simulink model "flightControlSystem"  (R2022b)
settings: Solver=ode3  StartTime=0  StopTime=TFinal  FixedStep=Ts  RelTol=1e-3  EnableMultiTasking=on
model workspace (MAT data in the model file):
  D_gain = 0.03
  I_gain = 1.9
  PD_gain = 4e-05
  P_gain = 6
  case0_gain = 0.999
  en = 0.4
  kado_delay = 20
  last_gain = 0.0008
  ririku = 400
  start = 1400
undefined symbols (not defined in the file): codertarget, Controller, DiscIntNeverNeededParam, Discrete, Estimator, g, gray, init, Sensors, Time, Ts, var_acc_angle_N, var_bias_gyr_N, var_gyro_p_N, Vehicle
libraries: simulink x80, visionstatistics x8, sldvlib x7, slpidlib x4, ctrlSharedLib x4, sharedtransform x3, dspstat3 x2, parrotlib x1
(part 1 of 3)
settings Model: ExtModeTrigDuration=80  Creator=The MathWorks, Inc.  LastModifiedBy=yasuh
settings SolverCC: ZeroCrossControl=DisableAll  AlgebraicLoopSolver=TrustRegion
settings DataIOCC: LimitDataPoints=on  SaveFormat=StructureWithTime  SaveOutput=off  DSMLogging=off  SaveTime=off  ReturnWorkspaceOutputs=off
settings OptimizationCC: BlockReduction=off  EnhancedBackFolding=on  PassReuseOutputArgsThreshold=0  MaxStackSize=64  OptimizeBlockOrder=speed  DifferentSizesBufferReuse=on  OptimizationCustomize=off
settings DebuggingCC: AlgebraicLoopMsg=none  ParameterPrecisionLossMsg=none  ParameterTunabilityLossMsg=error  BusObjectLabelMismatch=error  PregeneratedLibrarySubsystemCodeDiagnostic=none  SFUnexpectedBacktrackingDiag=warning  SFNoUnconditionalDefaultTransitionDiag=warning  SFExecutionAtInitializationDiag=none  SFMachineParentedDataDiag=warning  ArithmeticOperatorsInVariantConditions=warning
settings HardwareCC: ProdBitPerPointer=32  ProdBitPerSizeT=32  ProdBitPerPtrDiffT=32  ProdLargestAtomicInteger=Long  ProdWordSize=32  ProdHWDeviceType=ARM Compatible->ARM 9  UseEmbeddedCoderFeatures=off  UseSimulinkCoderFeatures=off
settings ModelReferenceCC: EnableRefExpFcnMdlSchedulingChecks=on  ModelReferenceNumInstancesAllowed=Single  PropagateSignalLabelsOutOfModel=off
settings SFSimCC: SimUseLocalCustomCode=off  MATLABDynamicMemAlloc=off  CustomCodeUndefinedFunction=UseInterfaceOnly
settings RTWCC: Description=Embedded Coder  SystemTargetFile=ert.tlc  HardwareBoard=PARROT Mambo  TLCOptions=-aInlineSetEventsForThisBaseRateFcn=TLC_FALSE -aSuppressMultiTaskScheduler=TLC_FALSE -aRateBasedStepFcn=1  TemplateMakefile=ert_default_tmf  RTWUseLocalCustomCode=off  Toolchain=Sourcery G++ Lite GNU Toolchain for Drones  DLArmComputeVersion=19.05
settings CodeAppCC: ForceParamTrailComments=on  MaxIdLength=63  OperatorAnnotations=on
settings ERTTargetCC: CombineOutputUpdateFcns=off  ERTCustomFileBanners=off  SupportContinuousTime=on  SupportNonInlinedSFcns=on  RemoveResetFunc=off  ModelStepFunctionPrototypeControlCompliant=off
settings ConfigComp: CovMetricSettings=dw  CovSaveCumulativeToWorkspaceVar=on  CovSaveSingleToWorkspaceVar=on  CovExternalEMLEnable=off  CovSFcnEnable=off

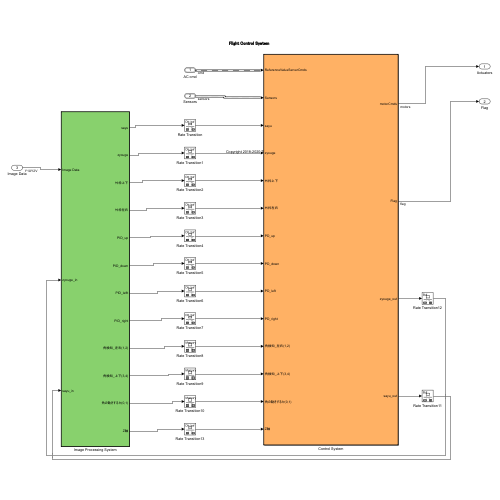
[thumbnail: Simulink's stored preview of the top-level diagram]
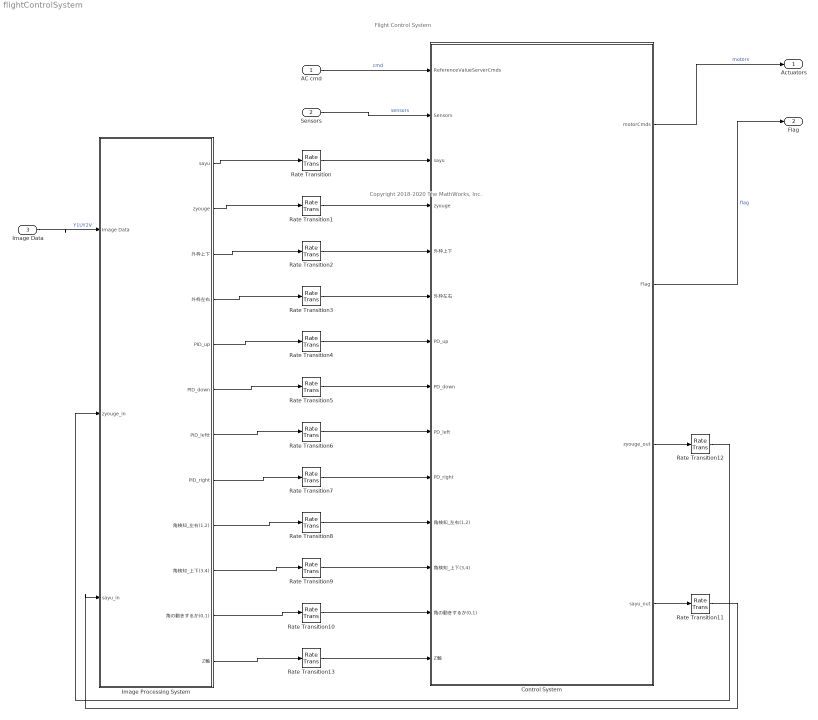
== system flightControlSystem ==
  note: Copyright 2018-2020 The MathWorks, Inc.
  note: Flight Control System
  AC cmd : Inport  OutDataTypeStr=Bus: CommandBus  BusOutputAsStruct=on
  Sensors : Inport  Port=2  OutDataTypeStr=Bus: SensorsBus  BusOutputAsStruct=on
  Image Data : Inport  Tag=IP_IN  InitFcn=codertarget.parrot.internal.inportCallback(gcb);  Port=3  OutDataTypeStr=uint8  PortDimensions=[4 9600]  BusOutputAsStruct=on
  Control System : Subsystem  InitFcn=codertarget.parrot.internal.fcsSubsystemCallback(gcb);  TreatAsAtomicUnit=on  SystemSampleTime=Ts
  Image Processing System : Subsystem  Tag=IP_SUB  InitFcn=codertarget.parrot.internal.ipSubsystemCallback(gcb);  TreatAsAtomicUnit=on  SystemSampleTime=40*Ts  RTWFcnName=ImageFunction
      settings: RTWSystemCode=Inline  RTWFcnNameOpts=User specified
  Rate Transition{,1..13} (14 alike) : RateTransition  Deterministic=off
  Actuators : Outport  OutDataTypeStr=single  PortDimensions=4  VectorParamsAs1DForOutWhenUnconnected=off
  Flag : Outport  Port=2  OutDataTypeStr=uint8  PortDimensions=1  VectorParamsAs1DForOutWhenUnconnected=off
  wires:
  AC cmd/1 -> Control System/1(ReferenceValueServerCmds)  "cmd"
  Control System/1(motorCmds) -> Actuators/1  "motors"
  Sensors/1 -> Control System/2(Sensors)  "sensors"
  Control System/2(Flag) -> Flag/1  "flag"
  Image Data/1 -> Image Processing System/1(Image Data)  "Y1UY2V"
  Image Processing System/1(sayu) -> Rate Transition/1
  Rate Transition/1 -> Control System/3(sayu)
  Image Processing System/2(zyouge) -> Rate Transition1/1
  Rate Transition1/1 -> Control System/4(zyouge)
  Image Processing System/3(外枠上下) -> Rate Transition2/1
  Image Processing System/4(外枠左右) -> Rate Transition3/1
  Rate Transition2/1 -> Control System/5(外枠上下)
  Rate Transition3/1 -> Control System/6(外枠左右)
  Image Processing System/5(PID_up) -> Rate Transition4/1
  Image Processing System/6(PID_down) -> Rate Transition5/1
  Rate Transition4/1 -> Control System/7(PD_up)
  Rate Transition5/1 -> Control System/8(PD_down)
  Image Processing System/7(PID_leftt) -> Rate Transition6/1
  Image Processing System/8(PID_right) -> Rate Transition7/1
  Rate Transition6/1 -> Control System/9(PD_left)
  Rate Transition7/1 -> Control System/10(PD_right)
  Image Processing System/11(角の動きするか(0,1)) -> Rate Transition10/1
  Rate Transition10/1 -> Control System/13(角の動きするか(0,1))
  Image Processing System/10(角検知_上下(3,4)) -> Rate Transition9/1
  Image Processing System/9(角検知_左右(1,2)) -> Rate Transition8/1
  Rate Transition9/1 -> Control System/12(角検知_上下(3,4))
  Rate Transition8/1 -> Control System/11(角検知_左右(1,2))
  Control System/3(zyouge_out) -> Rate Transition12/1
  Control System/4(sayu_out) -> Rate Transition11/1
  Rate Transition12/1 -> Image Processing System/2(zyouge_in)
  Rate Transition11/1 -> Image Processing System/3(sayu_in)
  Rate Transition13/1 -> Control System/14(Z軸)
  Image Processing System/12(Z軸) -> Rate Transition13/1

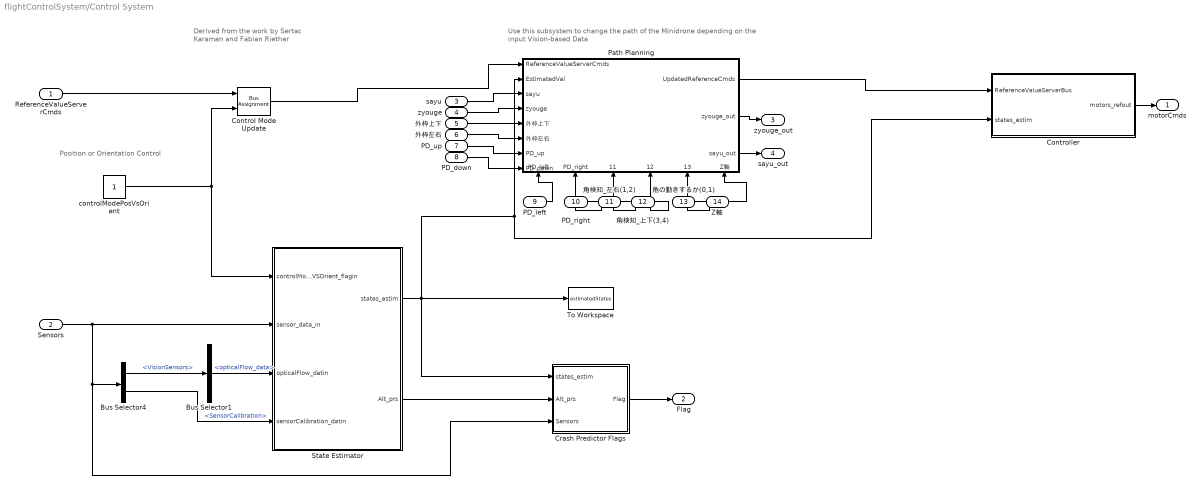
== system flightControlSystem/Control System ==
  note: Position or Orientation Control
  note: Use this subsystem to change the path of the
      | Minidrone depending on the input Vision-based
      | Data
  note: Derived from the work by Sertac
      | Karaman and Fabian Riether
  ReferenceValueServerCmds : Inport  OutDataTypeStr=Bus: CommandBus
  Sensors : Inport  Port=2  OutDataTypeStr=Bus: SensorsBus  BusOutputAsStruct=on
  sayu : Inport  Port=3
  zyouge : Inport  Port=4
  外枠上下 : Inport  Port=5
  外枠左右 : Inport  Port=6
  PD_up : Inport  Port=7
  PD_down : Inport  Port=8
  PD_left : Inport  Port=9
  PD_right : Inport  Port=10
  角検知_左右(1,2) : Inport  Port=11
  角検知_上下(3,4) : Inport  Port=12
  角の動きするか(0,1) : Inport  Port=13
  Z軸 : Inport  Port=14
  Bus Selector1 : BusSelector  OutputSignals=opticalFlow_data
  Bus Selector4 : BusSelector  OutputSignals=VisionSensors,SensorCalibration
  Control Mode Update : BusAssignment  AssignedSignals=controlModePosVSOrient
  Controller : Subsystem
  Crash Predictor Flags : Subsystem
  Path Planning : Subsystem
      settings: PortSchema="{\"entries\":[{\"content\":{\"sides\":[{\"content\":{\"connectorIds\":[\"In1\",\"In2\",\"In3\",\"In4\",\"In5\",\"In6\",\"In7\",\"In8\"]},\"type\":\"ConnectorPlacement.EquallySpacedRectSide\",\"uuid\":\"efe67c61-e99a-4cd7-b5d7-47091d682307\"},{\"content\":{\"connectorIds\":[\"Out1\",\"Out2\",\"Out3\"],\"side\":\"RIGHT\"},\"type\":\"ConnectorPlacement.EquallySpacedRectSide\",\"uuid\":\"b5496404-cc03-4446-9fbd-bd02e24f55c4\"},{\"content\":{\"connectorIds\":[],\"side\":\"TOP\"},\"type\":\"ConnectorPlacement.EquallySpacedRectSide\",\"uuid\":\"cc2bfd9b-f440-461f-8dfc-c1236b38a8d6\"},{\"content\":{\"connectorIds\":[\"In9\",\"In10\",\"In11\",\"In12\",\"In13\",\"In14\"],\"side\":\"BOTTOM\"},\"type\":\"ConnectorPlacement.EquallySpacedRectSide\",\"uuid\":\"b1dd3da0-6104-42b8-85e5-4e9639fd54d3\"}]},\"type\":\"ConnectorPlacement.EquallySpacedConnector\",\"uuid\":\"29da74a2-0098-4abc-a5c4-0db84ec285cd\"}],\"packageUris\":[\"http://schema.mathworks.com/mf0/Connector/R2020b\"],\"version\":\"1.0\"}"
  State Estimator : Subsystem
  To Workspace : ToWorkspace  VariableName=estimatedStates  SaveFormat=Structure With Time  SampleTime=-1
  controlModePosVsOrient : Constant  OutDataTypeStr=boolean
  motorCmds : Outport  VectorParamsAs1DForOutWhenUnconnected=off
  Flag : Outport  Port=2  VectorParamsAs1DForOutWhenUnconnected=off
  zyouge_out : Outport  Port=3  VectorParamsAs1DForOutWhenUnconnected=off
  sayu_out : Outport  Port=4  VectorParamsAs1DForOutWhenUnconnected=off
  wires:
  ReferenceValueServerCmds/1 -> Control Mode Update/1
  Bus Selector1/1 -> State Estimator/3(opticalFlow_datin)  "<opticalFlow_data>"
  Bus Selector4/2 -> State Estimator/4(sensorCalibration_datin)  "<SensorCalibration>"
  Path Planning/1(UpdatedReferenceCmds) -> Controller/1(ReferenceValueServerBus)
  Bus Selector4/1 -> Bus Selector1/1  "<VisionSensors>"
  sayu/1 -> Path Planning/3(sayu)
  Crash Predictor Flags/1(Flag) -> Flag/1
  Control Mode Update/1 -> Path Planning/1(ReferenceValueServerCmds)
  controlModePosVsOrient/1 -> State Estimator/1(controlModePosVSOrient_flagin), Control Mode Update/2
  Controller/1(motors_refout) -> motorCmds/1
  Sensors/1 -> State Estimator/2(sensor_data_in), Crash Predictor Flags/3(Sensors), Bus Selector4/1
  State Estimator/1(states_estim) -> Controller/2(states_estim), Path Planning/2(EstimatedVal), To Workspace/1, Crash Predictor Flags/1(states_estim)
  State Estimator/2(Alt_prs) -> Crash Predictor Flags/2(Alt_prs)
  zyouge/1 -> Path Planning/4(zyouge)
  外枠上下/1 -> Path Planning/5(外枠上下)
  外枠左右/1 -> Path Planning/6(外枠左右)
  PD_up/1 -> Path Planning/7(PD_up)
  PD_down/1 -> Path Planning/8(PD_down)
  PD_left/1 -> Path Planning/9(PD_left)
  PD_right/1 -> Path Planning/10(PD_right)
  角検知_左右(1,2)/1 -> Path Planning/11(角検知_左右(1,2))
  角検知_上下(3,4)/1 -> Path Planning/12(角検知_上下(3,4))
  角の動きするか(0,1)/1 -> Path Planning/13(角の動きするか(0,1))
  Path Planning/2(zyouge_out) -> zyouge_out/1
  Path Planning/3(sayu_out) -> sayu_out/1
  Z軸/1 -> Path Planning/14(Z軸)

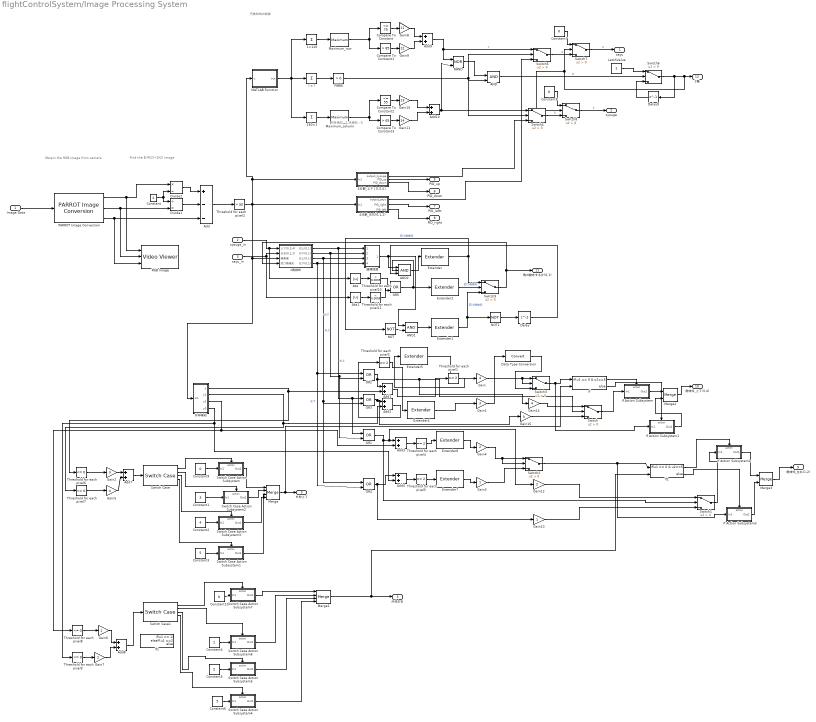
== system flightControlSystem/Image Processing System ==
  note: 円を検知：1
      | 　未検知：0
  note: 円検知時の制御
  note: Find the B-(R/2)-(G/2) image
  note: Obtain the RGB image from camera
  Image Data : Inport
  zyouge_in : Inport  Port=2
  sayu_in : Inport  Port=3
  160×1 : Sum  Inputs=+  CollapseMode=Specified dimension  CollapseDim=2
  1×120 : Sum  Inputs=+  CollapseMode=Specified dimension
  4分割_上下（0,3,4） : Subsystem
  4分割_左右(0,1,2) : Subsystem
  4角検知 : Subsystem
  AND : Logic  IconShape=distinctive  AllPortsSameDT=off  OutDataTypeStr=boolean
  AND1 : Logic  IconShape=distinctive  AllPortsSameDT=off  OutDataTypeStr=boolean
  AND2 : Logic  Inputs=3  IconShape=distinctive  AllPortsSameDT=off  OutDataTypeStr=boolean
  Abs : Abs  SaturateOnIntegerOverflow=off
  Abs1 : Abs  SaturateOnIntegerOverflow=off
  Add : Sum  Inputs=+--
  Add{1..4,9..10} (6 alike) : Sum
  Add7 : Sum  OutDataTypeStr=double
  Add8 : Sum  OutDataTypeStr=double
  Compare To Constant : simulink/Logic and Bit Operations/Compare To Constant  relop=<=  const=75  OutDataTypeStr=boolean
  Compare To Constant1 : simulink/Logic and Bit Operations/Compare To Constant  relop=>  const=85  OutDataTypeStr=boolean
  Compare To Constant2 : simulink/Logic and Bit Operations/Compare To Constant  relop=<=  const=55  OutDataTypeStr=boolean
  Compare To Constant3 : simulink/Logic and Bit Operations/Compare To Constant  relop=>  const=65  OutDataTypeStr=boolean
  Constant : Constant  Value=2
  Constant1 : Constant  Value=3
  Constant{7..10} (4 alike) : Constant  Value=0
  Constant2 : Constant  Value=4
  Constant3 : Constant  Value=5
  Constant4 : Constant
  Constant5 : Constant  Value=2
  Constant6 : Constant  Value=5
  Data Type Conversion : DataTypeConversion  SaturateOnIntegerOverflow=off  RndMeth=Floor
  Delay : Delay
  Delay9 : Delay  DelayLength=1
  Divide1 : Product  Inputs=/*
  Divide2 : Product  Inputs=*/
  Extender : sldvlib/Temporal Operators/Extender  reset=off  ext_type=Finite  out_hold=30
  Extender1 : sldvlib/Temporal Operators/Extender  reset=off  ext_type=Finite  out_hold=20
  Extender2 : sldvlib/Temporal Operators/Extender  reset=off  ext_type=Finite  out_hold=30
  Extender{4..7} (4 alike) : sldvlib/Temporal Operators/Extender  reset=off  ext_type=Finite  out_hold=kado_delay
  Gain : Gain  Gain=4
  Gain1 : Gain  Gain=3
  Gain10 : Gain  Gain=13
  Gain11 : Gain  Gain=14
  Gain12 : Gain  Gain=2
  Gain13 : Gain
  Gain14 : Gain  Gain=4
  Gain15 : Gain  Gain=3
  Gain2 : Gain  Gain=3
  Gain3 : Gain
  Gain4 : Gain  Gain=2
  Gain5 : Gain  Gain=4
  Gain6 : Gain
  Gain7 : Gain  Gain=2
  Gain8 : Gain  Gain=11
  Gain9 : Gain  Gain=12
  If : If  NumInputs=2  IfExpression=u1 == 0 & u2==5
  If Action Subsystem : Subsystem  TreatAsAtomicUnit=on
  If Action Subsystem1 : Subsystem  TreatAsAtomicUnit=on
  If Action Subsystem2 : Subsystem  TreatAsAtomicUnit=on
  If Action Subsystem3 : Subsystem  TreatAsAtomicUnit=on
  If1 : If  IfExpression=u1 == 1  ElseIfExpressions=u1 ==2
  If2 : If  NumInputs=2  IfExpression=u1 == 0 & u2==5
  LatchValue : Constant
  MATLAB Function : MATLAB Function  TreatAsAtomicUnit=on
  Maximum_column : dspstat3/Maximum  operation=maximum  fcn=Index  indexBase=One  operateOver=Each column  Dimension=1  InputProcessing=Columns as channels (frame based)  reset=None  roiEnable=off  roiType=Rectangles  roiPortion=Entire ROI  roiOutput=Individual statistics for each ROI  roiFlag=off  roundingMode=Floor  overflowMode=off  accumDataTypeStr=Inherit: Same as product output  accumLastDataTypeStr=Inherit: Same as product output
      settings: LibrarySourceBlock=dsphdlsupportstat/Maximum
  Maximum_row : dspstat3/Maximum  operation=maximum  fcn=Index  indexBase=One  operateOver=Each row  Dimension=1  InputProcessing=Columns as channels (frame based)  reset=None  roiEnable=off  roiType=Rectangles  roiPortion=Entire ROI  roiOutput=Individual statistics for each ROI  roiFlag=off  roundingMode=Floor  overflowMode=off  accumDataTypeStr=Inherit: Same as product output  accumLastDataTypeStr=Inherit: Same as product output
      settings: LibrarySourceBlock=dsphdlsupportstat/Maximum
  Merge : Merge  Inputs=4
  Merge1 : Merge  Inputs=4
  Merge2 : Merge
  Merge3 : Merge
  NAND : Logic  Operator=NOR  IconShape=distinctive  AllPortsSameDT=off  OutDataTypeStr=boolean
  NOT : Logic  Operator=NOT  IconShape=distinctive  AllPortsSameDT=off  OutDataTypeStr=boolean
  NOT1 : Logic  Operator=NOT  IconShape=distinctive  AllPortsSameDT=off  OutDataTypeStr=boolean
  OR{1..5} (5 alike) : Logic  Operator=OR  IconShape=distinctive  AllPortsSameDT=off  OutDataTypeStr=boolean
  PARROT Image Conversion : parrotlib/PARROT Image Conversion  ImageFormat=RGB  R=on  Y=on  G=on  U=on  B=on  V=on
  RGB Image : VideoViewer  imagePorts=separate color signals  colormapValue=gray(256)  FigPos=[798.333333333333 546 354 271.333333333333]
  Switch : Switch  Criteria=u2 > Threshold  OutDataTypeStr=double  SaturateOnIntegerOverflow=off  InputSameDT=off
  Switch Case : SwitchCase  CaseConditions={0,3,4,7}
  Switch Case Action Subsystem : Subsystem  TreatAsAtomicUnit=on
  Switch Case Action Subsystem1 : Subsystem  TreatAsAtomicUnit=on
  Switch Case Action Subsystem2 : Subsystem  TreatAsAtomicUnit=on
  Switch Case Action Subsystem3 : Subsystem  TreatAsAtomicUnit=on
  Switch Case Action Subsystem4 : Subsystem  TreatAsAtomicUnit=on
  Switch Case Action Subsystem5 : Subsystem  TreatAsAtomicUnit=on
  Switch Case Action Subsystem6 : Subsystem  TreatAsAtomicUnit=on
  Switch Case Action Subsystem7 : Subsystem  TreatAsAtomicUnit=on
  Switch Case1 : SwitchCase  CaseConditions={0,1,2,3}
  Switch1 : Switch  Criteria=u2 > Threshold  OutDataTypeStr=double  SaturateOnIntegerOverflow=off  InputSameDT=off
  Switch2 : Switch  Criteria=u2 > Threshold  OutDataTypeStr=double  SaturateOnIntegerOverflow=off  InputSameDT=off
  Switch3 : Switch  Criteria=u2 > Threshold  OutDataTypeStr=double  SaturateOnIntegerOverflow=off
  Switch{4..9} (6 alike) : Switch  Criteria=u2 > Threshold  SaturateOnIntegerOverflow=off  InputSameDT=off
  Threshold for each pixel{1,3..5} (4 alike) : simulink/Logic and Bit Operations/Compare To Constant  relop===  const=2  OutDataTypeStr=boolean
  Threshold for each pixel10 : simulink/Logic and Bit Operations/Compare To Constant  relop=<  const=0.0005  OutDataTypeStr=boolean
  Threshold for each pixel11 : simulink/Logic and Bit Operations/Compare To Constant  relop=<  const=0.0005  OutDataTypeStr=boolean
  Threshold for each pixel2 : simulink/Logic and Bit Operations/Compare To Constant  relop=>  const=50  OutDataTypeStr=boolean
  Threshold for each pixel{6..9} (4 alike) : simulink/Logic and Bit Operations/Compare To Constant  relop=<=  const=0  OutDataTypeStr=boolean
  円検知 : simulink/Logic and Bit Operations/Compare To Constant  relop=>  const=0  OutDataTypeStr=boolean
  外枠検知 : Subsystem
  論理回路 : Subsystem
  １×１ : Sum  Inputs=+  CollapseDim=2  AccumDataTypeStr=double
  sayu : Outport  VectorParamsAs1DForOutWhenUnconnected=off
  zyouge : Outport  Port=2  VectorParamsAs1DForOutWhenUnconnected=off
  外枠上下 : Outport  Port=3
  外枠左右 : Outport  Port=4
  PID_up : Outport  Port=5
  PID_down : Outport  Port=6
  PID_leftt : Outport  Port=7
  PID_right : Outport  Port=8
  角検知_左右(1,2) : Outport  Port=9
  角検知_上下(3,4) : Outport  Port=10
  角の動きするか(0,1) : Outport  Port=11
  Z軸 : Outport  Port=12
  wires:
  Divide2/1 -> Add/1
  PARROT Image Conversion/3 -> RGB Image/3, Add/3
  PARROT Image Conversion/1 -> RGB Image/1, Divide2/1
  PARROT Image Conversion/2 -> RGB Image/2, Divide1/2
  Divide1/1 -> Add/2
  Constant/1 -> Divide1/1, Divide2/2
  Image Data/1 -> PARROT Image Conversion/1
  4分割_左右(0,1,2)/1(output_sayu) -> Switch5/3
  Threshold for each pixel2/1 -> 外枠検知/1(In1), 4角検知/3(画素値), 4分割_左右(0,1,2)/1(In1), MATLAB Function/1(u), 4分割_上下（0,3,4）/1(In1)
  4角検知/2(右下(0,1)) -> 論理回路/2(In2), OR2/2, OR1/2  "右下"
  4角検知/3(左上(0,1)) -> 論理回路/3(In3), OR4/1, OR3/2  "左上"
  4角検知/4(左下(0,1)) -> OR2/1, OR4/2, 論理回路/4(In4)  "左下"
  OR2/1 -> Gain14/1, Switch/2, Add1/1
  Threshold for each pixel1/1 -> Extender5/1
  OR1/1 -> Switch1/2, Gain12/1, Add3/1
  OR3/1 -> Gain15/1, Add2/1
  Threshold for each pixel3/1 -> Extender4/1
  Add4/1 -> Threshold for each pixel5/1
  OR4/1 -> Gain13/1, Add4/1
  Gain/1 -> Switch3/1, Switch3/2
  Add1/1 -> Threshold for each pixel1/1
  Add2/1 -> Threshold for each pixel3/1
  Threshold for each pixel4/1 -> Extender6/1
  Threshold for each pixel5/1 -> Extender7/1
  4角検知/1(右上(0,1)) -> 論理回路/1(In1), OR3/1, OR1/1  "右上"
  Extender4/1 -> Gain1/1
  Extender5/1 -> Gain/1
  Extender6/1 -> Gain4/1
  Extender7/1 -> Gain3/1
  外枠検知/1(y) -> Threshold for each pixel6/1, Add1/2
  Threshold for each pixel6/1 -> Gain2/1
  外枠検知/2(y1) -> Add2/2, Threshold for each pixel7/1
  Threshold for each pixel7/1 -> Gain5/1
  外枠検知/3(y2) -> Add3/2, Threshold for each pixel8/1
  Threshold for each pixel8/1 -> Gain6/1
  外枠検知/4(y3) -> Add4/2, Threshold for each pixel9/1
  Threshold for each pixel9/1 -> Gain7/1
  Merge/1 -> If/2, 外枠上下/1
  Gain2/1 -> Add7/1
  Gain5/1 -> Add7/2
  Add7/1 -> Switch Case/1
  Constant1/1 -> Switch Case Action Subsystem2/1(In1)
  Switch Case Action Subsystem2/1(Out1) -> Merge/2
  Constant2/1 -> Switch Case Action Subsystem3/1(In1)
  Switch Case Action Subsystem3/1(Out1) -> Merge/4
  Constant3/1 -> Switch Case Action Subsystem1/1(In1)
  Switch Case Action Subsystem1/1(Out1) -> Merge/3
  Merge1/1 -> If2/2, 外枠左右/1
  Gain6/1 -> Add8/1
  Gain7/1 -> Add8/2
  Add8/1 -> Switch Case1/1
  Constant5/1 -> Switch Case Action Subsystem5/1(In1)
  Constant6/1 -> Switch Case Action Subsystem4/1(In1)
  Switch Case Action Subsystem4/1(Out1) -> Merge1/4
  Switch Case Action Subsystem5/1(Out1) -> Merge1/3
  4分割_上下（0,3,4）/2(PID_up) -> PID_up/1
  4分割_上下（0,3,4）/3(PID_down) -> PID_down/1
  4分割_左右(0,1,2)/2(PID_right) -> PID_leftt/1
  4分割_左右(0,1,2)/3(PID_left) -> PID_right/1
  sayu_in/1 -> Abs1/1, 4角検知/2(左右(0,1,2))
  zyouge_in/1 -> Abs/1, 4角検知/1(上下(0,3,4))
  Add/1 -> Threshold for each pixel2/1
  AND/1 -> Switch6/2  "Z"
  1×120/1 -> Maximum_row/1
  Gain11/1 -> Add10/2
  4分割_上下（0,3,4）/1(output_zyouge) -> Switch4/3
  Maximum_row/1 -> Compare To Constant1/1, Compare To Constant/1
  １×１/1 -> 円検知/1
  160×1/1 -> Maximum_column/1
  Compare To Constant2/1 -> Gain10/1
  Gain9/1 -> Add9/2
  Gain10/1 -> Add10/1
  Add10/1 -> NAND/2, Switch4/1
  MATLAB Function/1(out) -> 1×120/1, １×１/1, 160×1/1
  NAND/1 -> AND/1
  Compare To Constant3/1 -> Gain11/1
  Switch8/1 -> zyouge/1  "X"
  Add9/1 -> Switch5/1, NAND/1  "Y"
  Compare To Constant1/1 -> Gain9/1
  Compare To Constant/1 -> Gain8/1
  Gain8/1 -> Add9/1
  円検知/1 -> Switch5/2, Switch4/2, AND/2
  Maximum_column/1 -> Compare To Constant2/1, Compare To Constant3/1
  Switch7/1 -> sayu/1  "X"
  Switch6/1 -> Switch8/2, Switch7/2, Z軸/1, Delay9/1
  LatchValue/1 -> Switch6/1
  Delay9/1 -> Switch6/3
  Switch5/1 -> Switch7/3  "X"
  Constant7/1 -> Switch7/1
  Constant8/1 -> Switch8/1
  Switch4/1 -> Switch8/3  "X"
  Switch3/1 -> If/1, If Action Subsystem1/1(In1)
  Switch Case/2 -> Switch Case Action Subsystem2/Action
  Switch Case/3 -> Switch Case Action Subsystem3/Action
  Switch Case/4 -> Switch Case Action Subsystem1/Action
  Switch Case/1 -> Switch Case Action Subsystem/Action
  Constant9/1 -> Switch Case Action Subsystem/1(In1)
  Switch Case Action Subsystem/1(Out1) -> Merge/1
  Switch Case1/2 -> Switch Case Action Subsystem6/Action
  Switch Case1/3 -> Switch Case Action Subsystem5/Action
  Switch Case1/4 -> Switch Case Action Subsystem4/Action
  Switch Case1/1 -> Switch Case Action Subsystem7/Action
  Constant10/1 -> Switch Case Action Subsystem7/1(In1)
  Switch Case Action Subsystem7/1(Out1) -> Merge1/1
  Constant4/1 -> Switch Case Action Subsystem6/1(In1)
  Switch Case Action Subsystem6/1(Out1) -> Merge1/2
  If/1 -> If Action Subsystem/Action
  Switch/1 -> If Action Subsystem/1(In1)
  If Action Subsystem/1(Out1) -> Merge2/1
  If/2 -> If Action Subsystem1/Action
  If Action Subsystem1/1(Out1) -> Merge2/2
  Merge2/1 -> 角検知_上下(3,4)/1
  If2/1 -> If Action Subsystem2/Action
  Switch1/1 -> If Action Subsystem2/1(In1)
  Add3/1 -> Threshold for each pixel4/1
  Gain4/1 -> Switch2/1, Switch2/2
  If2/2 -> If Action Subsystem3/Action
  If Action Subsystem2/1(Out1) -> Merge3/1
  If Action Subsystem3/1(Out1) -> Merge3/2
  Switch2/1 -> If Action Subsystem3/1(In1), If2/1
  Gain3/1 -> Switch2/3
  Merge3/1 -> 角検知_左右(1,2)/1
  Gain1/1 -> Data Type Conversion/1
  Data Type Conversion/1 -> Switch3/3
  Gain12/1 -> Switch1/1
  Gain13/1 -> Switch1/3
  Gain14/1 -> Switch/1
  Gain15/1 -> Switch/3
  Abs/1 -> Threshold for each pixel10/1
  Abs1/1 -> Threshold for each pixel11/1
  Switch9/1 -> 4角検知/4(四つ角検知), 角の動きするか(0,1)/1
  Threshold for each pixel10/1 -> OR5/1
  Threshold for each pixel11/1 -> OR5/2
  OR5/1 -> Extender2/1, AND2/2
  論理回路/1(Out1) -> AND2/1, AND1/1
  Extender/1 -> Switch9/1, NOT/1  "四つ角検知"
  NOT/1 -> AND1/2
  AND1/1 -> Extender1/1
  Extender1/1 -> NOT1/1, Switch9/3  "四つ角検知"
  Extender2/1 -> Switch9/2  "四つ角検知"
  AND2/1 -> Extender/1
  NOT1/1 -> Delay/1
  Delay/1 -> AND2/3

== system flightControlSystem/Control System/Controller ==
  In Bus Element1 : Inport  PortName=ReferenceValueServerBus  Element=controlModePosVSOrient
  In Bus Element : Inport  PortName=ReferenceValueServerBus  Element=pos_ref
  In Bus Element5 : Inport  PortName=ReferenceValueServerBus  Element=pos_ref
  In Bus Element2 : Inport  PortName=ReferenceValueServerBus  Element=orient_ref
  In Bus Element6 : Inport  PortName=ReferenceValueServerBus  Element=orient_ref
  In Bus Element3 : Inport  PortName=ReferenceValueServerBus  Element=takeoff_flag
  states_estim : Inport  Port=2
  Altitude Controller : Subsystem
  Attitude Controller : Subsystem
  ControlMixer : Subsystem
  Position Controller : Subsystem
  Selector : Selector  InputPortWidth=3  IndexOptions=Index vector (dialog)  Indices=3  OutputSizes=1
  Selector1 : Selector  InputPortWidth=3  IndexOptions=Index vector (dialog)  Indices=[1 2]  OutputSizes=1
  Selector2 : Selector  InputPortWidth=3  IndexOptions=Index vector (dialog)  Indices=[2 3]  OutputSizes=1
  Selector3 : Selector  InputPortWidth=3  IndexOptions=Index vector (dialog)  Indices=1  OutputSizes=1
  Switch_refAtt : Switch  Criteria=u2 > Threshold  SaturateOnIntegerOverflow=off  InputSameDT=off
  Yaw Controller : Subsystem
  states_estim1 : InportShadow  Port=2
  states_estim2 : InportShadow  Port=2
  states_estim3 : InportShadow  Port=2
  thrustsToMotorCommands : Subsystem
  motors_refout : Outport  VectorParamsAs1DForOutWhenUnconnected=off
  wires:
  thrustsToMotorCommands/1(motors_cmdout) -> motors_refout/1
  In Bus Element5/1 -> Selector/1
  states_estim3/1 -> Position Controller/2(states_estim)
  In Bus Element6/1 -> Selector2/1
  Selector3/1 -> Yaw Controller/1(yaw_ref)
  In Bus Element/1 -> Selector1/1
  ControlMixer/1(thrusts_refout) -> thrustsToMotorCommands/1(thrusts_refin)
  Selector2/1 -> Switch_refAtt/3
  Altitude Controller/1(altitude_cmd) -> ControlMixer/4(totalThrust)
  Selector1/1 -> Position Controller/1(posXY)  "pos"
  states_estim1/1 -> Altitude Controller/1(states_estim)
  Selector/1 -> Altitude Controller/2(PosZ)
  In Bus Element3/1 -> Altitude Controller/3(takeoff_flag)
  states_estim/1 -> Yaw Controller/2(states_estim)
  Position Controller/1(pitch_roll_cmd) -> Switch_refAtt/1
  In Bus Element2/1 -> Selector3/1
  In Bus Element1/1 -> Switch_refAtt/2
  Switch_refAtt/1 -> Attitude Controller/1(refAttitude)
  states_estim2/1 -> Attitude Controller/2(states_estim)
  Attitude Controller/1(tau_pitch) -> ControlMixer/1(tau_pitch)
  Attitude Controller/2(tau_roll) -> ControlMixer/2(tau_roll)
  Yaw Controller/1(tau_yaw) -> ControlMixer/3(tau_yaw)

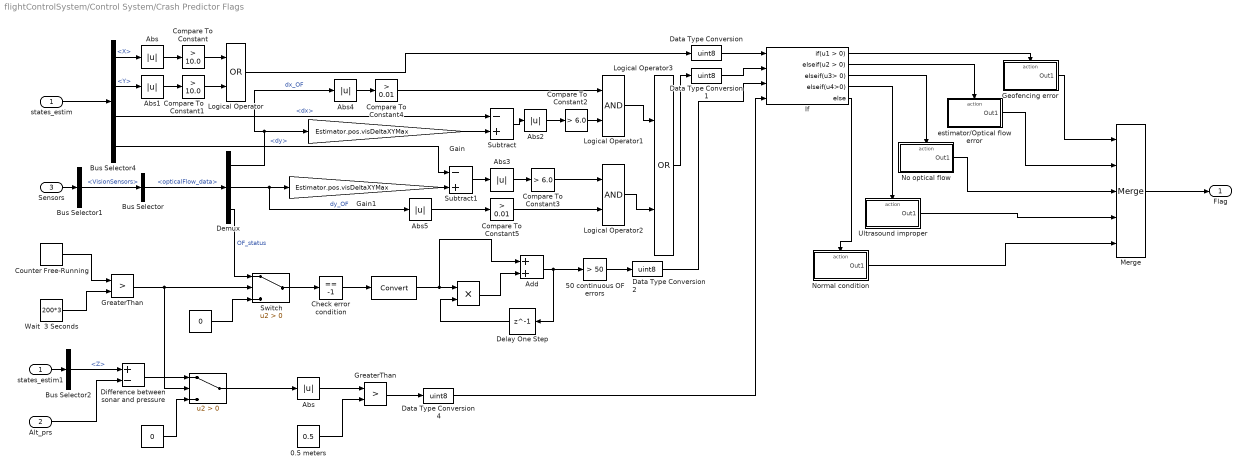
== system flightControlSystem/Control System/Crash Predictor Flags ==
  states_estim : Inport
  Alt_prs : Inport  Port=2
  Sensors : Inport  Port=3
  " " : Constant  Value=0
  "  " : Product  Inputs=**
  "   " : DataTypeConversion  SaturateOnIntegerOverflow=off  RndMeth=Floor
  "    " : Constant  Value=0  OutDataTypeStr=single
  "         " : Switch  Criteria=u2 > Threshold  SaturateOnIntegerOverflow=off  InputSameDT=off
  0.5 meters : Constant  Value=0.5
  "50 continuous OF errors " : simulink/Logic and Bit Operations/Compare To Constant  relop=>  const=50  OutDataTypeStr=boolean
  Abs{,1..5} (6 alike) : Abs  SaturateOnIntegerOverflow=off
  "Abs  " : Abs  SaturateOnIntegerOverflow=off
  Add : Sum
  Bus Selector : BusSelector  OutputSignals=opticalFlow_data
  Bus Selector1 : BusSelector  OutputSignals=VisionSensors
  Bus Selector2 : BusSelector  OutputSignals=Z
  Bus Selector4 : BusSelector  OutputSignals=X,Y,dx,dy
  Check error condition : simulink/Logic and Bit Operations/Compare To Constant  relop===  const=-1  OutDataTypeStr=boolean
  Compare To Constant : simulink/Logic and Bit Operations/Compare To Constant  relop=>  const=10.0  OutDataTypeStr=boolean
  Compare To Constant1 : simulink/Logic and Bit Operations/Compare To Constant  relop=>  const=10.0  OutDataTypeStr=boolean
  Compare To Constant2 : simulink/Logic and Bit Operations/Compare To Constant  relop=>  const=6.0  OutDataTypeStr=boolean
  Compare To Constant3 : simulink/Logic and Bit Operations/Compare To Constant  relop=>  const=6.0  OutDataTypeStr=boolean
  Compare To Constant4 : simulink/Logic and Bit Operations/Compare To Constant  relop=>  const=0.01  OutDataTypeStr=boolean
  Compare To Constant5 : simulink/Logic and Bit Operations/Compare To Constant  relop=>  const=0.01  OutDataTypeStr=boolean
  Counter Free-Running : simulink/Sources/Counter Free-Running  NumBits=32  tsamp=-1
  Data Type Conversion{,1..2,4} (4 alike) : DataTypeConversion  OutDataTypeStr=uint8  RndMeth=Nearest  SaturateOnIntegerOverflow=off
  Delay One Step : Delay  DelayLength=1
  Demux : Demux  Outputs=3
  Difference between sonar and pressure : Sum  Inputs=+-
  Gain : Gain  Gain=Estimator.pos.visDeltaXYMax
  Gain1 : Gain  Gain=Estimator.pos.visDeltaXYMax
  Geofencing error : Subsystem  TreatAsAtomicUnit=on
  GreaterThan : RelationalOperator  Operator=>  OutDataTypeStr=boolean  RndMeth=Simplest  InputSameDT=off
  "GreaterThan  " : RelationalOperator  Operator=>  OutDataTypeStr=boolean  RndMeth=Simplest  InputSameDT=off
  If : If  NumInputs=4  ElseIfExpressions=u2 > 0, u3> 0,u4>0
  Logical Operator : Logic  Operator=OR  AllPortsSameDT=off
  Logical Operator1 : Logic  AllPortsSameDT=off  OutDataTypeStr=boolean
  Logical Operator2 : Logic  AllPortsSameDT=off  OutDataTypeStr=boolean
  Logical Operator3 : Logic  Operator=OR  AllPortsSameDT=off
  Merge : Merge  Inputs=5  InitialOutput=0
  "No optical flow " : Subsystem  TreatAsAtomicUnit=on
  Normal condition : Subsystem  TreatAsAtomicUnit=on
  Subtract : Sum  Inputs=-+
  Subtract1 : Sum  Inputs=-+
  Switch : Switch  Criteria=u2 > Threshold  SaturateOnIntegerOverflow=off  InputSameDT=off
  Ultrasound improper : Subsystem  TreatAsAtomicUnit=on
  Wait  3 Seconds : Constant  Value=200*3
  estimator/Optical flow error : Subsystem  TreatAsAtomicUnit=on
  states_estim1 : InportShadow
  Flag : Outport  VectorParamsAs1DForOutWhenUnconnected=off
  wires:
  Bus Selector4/1 -> Abs/1  "<X>"
  states_estim/1 -> Bus Selector4/1
  Bus Selector4/2 -> Abs1/1  "<Y>"
  Compare To Constant/1 -> Logical Operator/1
  Compare To Constant1/1 -> Logical Operator/2
  Abs/1 -> Compare To Constant/1
  Abs1/1 -> Compare To Constant1/1
  Logical Operator/1 -> Data Type Conversion/1
  Bus Selector/1 -> Demux/1  "<opticalFlow_data>"
  Demux/1 -> Abs4/1, Gain/1  "dx_OF"
  Demux/2 -> Gain1/1, Abs5/1  "dy_OF"
  Bus Selector4/3 -> Subtract/1  "<dx>"
  Subtract/1 -> Abs2/1
  Subtract1/1 -> Abs3/1
  Abs2/1 -> Compare To Constant2/1
  Abs3/1 -> Compare To Constant3/1
  Compare To Constant5/1 -> Logical Operator2/2
  Abs4/1 -> Compare To Constant4/1
  Abs5/1 -> Compare To Constant5/1
  Compare To Constant3/1 -> Logical Operator2/1
  Logical Operator1/1 -> Logical Operator3/1
  Logical Operator2/1 -> Logical Operator3/2
  Logical Operator3/1 -> Data Type Conversion1/1
  Gain/1 -> Subtract/2
  Bus Selector4/4 -> Subtract1/1  "<dy>"
  Gain1/1 -> Subtract1/2
  Compare To Constant4/1 -> Logical Operator1/1
  Compare To Constant2/1 -> Logical Operator1/2
  Sensors/1 -> Bus Selector1/1
  Bus Selector1/1 -> Bus Selector/1  "<VisionSensors>"
  Merge/1 -> Flag/1
  If/1 -> Geofencing error/Action
  If/2 -> estimator/Optical flow error/Action
  If/5 -> Normal condition/Action
  Geofencing error/1(Out1) -> Merge/1
  estimator/Optical flow error/1(Out1) -> Merge/2
  Normal condition/1(Out1) -> Merge/5
  Data Type Conversion/1 -> If/1
  Data Type Conversion1/1 -> If/2
  Check error condition/1 -> "   "/1
  Demux/3 -> Switch/1  "OF_status"
  Delay One Step/1 -> "  "/2
  Add/1 -> Delay One Step/1, "50 continuous OF errors "/1
  "  "/1 -> Add/2
  "50 continuous OF errors "/1 -> Data Type Conversion2/1
  Data Type Conversion2/1 -> If/3
  "No optical flow "/1(Out1) -> Merge/3
  If/3 -> "No optical flow "/Action
  "   "/1 -> Add/1, "  "/1
  Counter Free-Running/1 -> GreaterThan/1
  Wait  3 Seconds/1 -> GreaterThan/2
  Switch/1 -> Check error condition/1
  " "/1 -> Switch/3
  "    "/1 -> "         "/3
  Difference between sonar and pressure/1 -> "         "/1
  Bus Selector2/1 -> Difference between sonar and pressure/1  "<Z>"
  GreaterThan/1 -> Switch/2, "         "/2
  "         "/1 -> "Abs  "/1
  "Abs  "/1 -> "GreaterThan  "/1
  0.5 meters/1 -> "GreaterThan  "/2
  Alt_prs/1 -> Difference between sonar and pressure/2
  "GreaterThan  "/1 -> Data Type Conversion4/1
  states_estim1/1 -> Bus Selector2/1
  Data Type Conversion4/1 -> If/4
  Ultrasound improper/1(Out1) -> Merge/4
  If/4 -> Ultrasound improper/Action

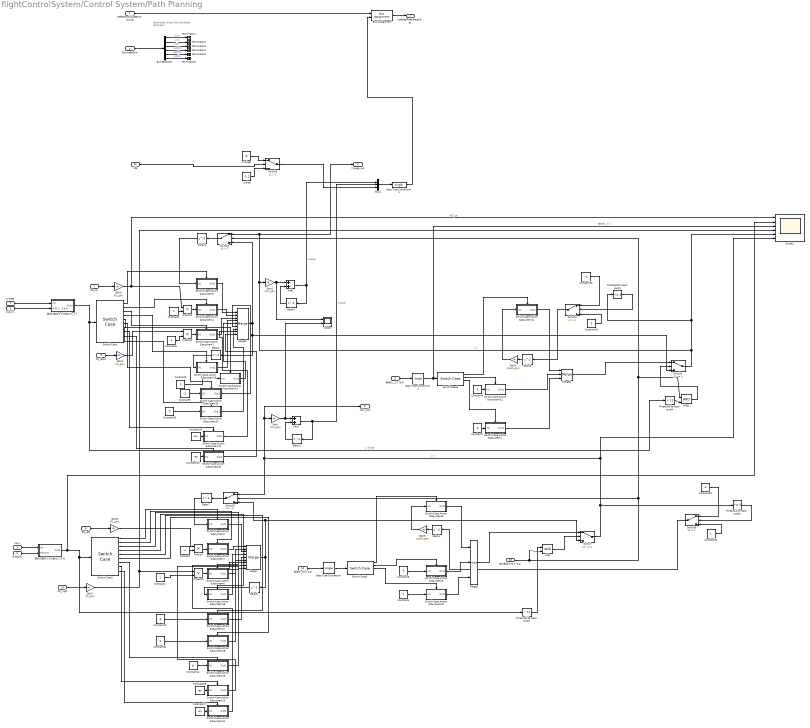
== system flightControlSystem/Control System/Path Planning ==
  note: Estimated values from the
      | State Estimator
  ReferenceValueServerCmds : Inport
  EstimatedVal : Inport  Port=2
  sayu : Inport  Port=3
  zyouge : Inport  Port=4
  外枠上下 : Inport  Port=5
  外枠左右 : Inport  Port=6
  PD_up : Inport  Port=7
  PD_down : Inport  Port=8
  PD_left : Inport  Port=9
  PD_right : Inport  Port=10
  角検知_左右(1,2) : Inport  Port=11
  角検知_上下(3,4) : Inport  Port=12
  角の動きするか(0,1) : Inport  Port=13
  Z軸 : Inport  Port=14
  AND : Logic  IconShape=distinctive  AllPortsSameDT=off  OutDataTypeStr=boolean
  AND1 : Logic  IconShape=distinctive  AllPortsSameDT=off  OutDataTypeStr=boolean
  Add1 : Sum
  Add2 : Sum
  Bus Selector1 : BusSelector  OutputSignals=X,Y,Z,yaw,pitch,roll
  Bus Assignment : BusAssignment  AssignedSignals=pos_ref
  Constant{,3,5,7,9..10,18,20} (8 alike) : Constant  Value=-1
  Constant{1..2,4,6,8,11,19,21} (8 alike) : Constant
  Constant12 : Constant  Value=0
  Constant13 : Constant  Value=0
  Constant14 : Constant  Value=en
  Constant15 : Constant  Value=-en
  Constant16 : Constant  Value=-en
  Constant17 : Constant  Value=en
  Data Type Conversion : DataTypeConversion  OutDataTypeStr=single  RndMeth=Nearest  SaturateOnIntegerOverflow=off
  Data Type Conversion1 : DataTypeConversion  OutDataTypeStr=single  SaturateOnIntegerOverflow=off  RndMeth=Floor
  Data Type Conversion2 : DataTypeConversion  OutDataTypeStr=single  RndMeth=Nearest  SaturateOnIntegerOverflow=off
  Delay1 : Delay  InitialCondition=0
  Delay2 : Delay
  Delay{3..4,6..7} (4 alike) : Delay  DelayLength=1
  Delay5 : Delay
  Delay8 : Delay  InitialCondition=0
  Gain : Gain  Gain=last_gain
  Gain1 : Gain  Gain=last_gain
  Gain{2,5..7} (4 alike) : Gain  Gain=PD_gain
  Gain3 : Gain  Gain=case0_gain
  Gain8 : Gain  Gain=case0_gain
  Merge : Merge  Inputs=9
  Merge1 : Merge  Inputs=9
  Merge2 : Merge  Inputs=3
  Merge3 : Merge  Inputs=3
  Mux1 : Mux  Inputs=3
  Product{,1..3} (4 alike) : Product
  Scope : Scope  NumInputPorts=2
  Scope1 : Scope  NumInputPorts=6
  Switch : Switch  Criteria=u2 ~= 0  Threshold=1  SaturateOnIntegerOverflow=off  InputSameDT=off
  Switch Case : SwitchCase  CaseConditions={5,3,4,10,6,8,0,13,14}
  Switch Case Action Subsystem1 : Subsystem  TreatAsAtomicUnit=on
  Switch Case Action Subsystem10 : Subsystem  TreatAsAtomicUnit=on
  Switch Case Action Subsystem11 : Subsystem  TreatAsAtomicUnit=on
  Switch Case Action Subsystem12 : Subsystem  TreatAsAtomicUnit=on
  Switch Case Action Subsystem13 : Subsystem  TreatAsAtomicUnit=on
  Switch Case Action Subsystem14 : Subsystem  TreatAsAtomicUnit=on
  Switch Case Action Subsystem15 : Subsystem  TreatAsAtomicUnit=on
  Switch Case Action Subsystem16 : Subsystem  TreatAsAtomicUnit=on
  Switch Case Action Subsystem17 : Subsystem  TreatAsAtomicUnit=on
  Switch Case Action Subsystem18 : Subsystem  TreatAsAtomicUnit=on
  Switch Case Action Subsystem19 : Subsystem  TreatAsAtomicUnit=on
  Switch Case Action Subsystem2 : Subsystem  TreatAsAtomicUnit=on
  Switch Case Action Subsystem20 : Subsystem  TreatAsAtomicUnit=on
  Switch Case Action Subsystem21 : Subsystem  TreatAsAtomicUnit=on
  Switch Case Action Subsystem22 : Subsystem  TreatAsAtomicUnit=on
  Switch Case Action Subsystem23 : Subsystem  TreatAsAtomicUnit=on
  Switch Case Action Subsystem24 : Subsystem  TreatAsAtomicUnit=on
  Switch Case Action Subsystem3 : Subsystem  TreatAsAtomicUnit=on
  Switch Case Action Subsystem4 : Subsystem  TreatAsAtomicUnit=on
  Switch Case Action Subsystem5 : Subsystem  TreatAsAtomicUnit=on
  Switch Case Action Subsystem6 : Subsystem  TreatAsAtomicUnit=on
  Switch Case Action Subsystem7 : Subsystem  TreatAsAtomicUnit=on
  Switch Case Action Subsystem8 : Subsystem  TreatAsAtomicUnit=on
  Switch Case Action Subsystem9 : Subsystem  TreatAsAtomicUnit=on
  Switch Case1 : SwitchCase  CaseConditions={5,1,2,15,3,6,0,11,12}
  Switch Case2 : SwitchCase  CaseConditions={0,1,2,5}
  Switch Case3 : SwitchCase  CaseConditions={0,3,4,}
  Switch1 : Switch  Criteria=u2 ~= 0  Threshold=1  SaturateOnIntegerOverflow=off  InputSameDT=off
  Switch{2..6} (5 alike) : Switch  Criteria=u2 > Threshold  SaturateOnIntegerOverflow=off  InputSameDT=off
  Terminator{1..6} (6 alike) : Terminator
  Threshold for each pixel1 : simulink/Logic and Bit Operations/Compare To Constant  relop=<=  const=0  OutDataTypeStr=boolean
  Threshold for each pixel2 : simulink/Logic and Bit Operations/Compare To Constant  relop=<  const=11  OutDataTypeStr=boolean
  Threshold for each pixel3 : simulink/Logic and Bit Operations/Compare To Constant  relop=<=  const=0  OutDataTypeStr=boolean
  Threshold for each pixel4 : simulink/Logic and Bit Operations/Compare To Constant  relop=<  const=13  OutDataTypeStr=boolean
  zValue : Constant  Value=-1.1
  zValue2 : Constant  Value=0
  最初の動きと4分割出力_上下 : Subsystem
  最初の動きと4分割出力_左右 : Subsystem
  UpdatedReferenceCmds : Outport  VectorParamsAs1DForOutWhenUnconnected=off
  zyouge_out : Outport  Port=2  VectorParamsAs1DForOutWhenUnconnected=off
  sayu_out : Outport  Port=3  VectorParamsAs1DForOutWhenUnconnected=off
  wires:
  Bus Assignment/1 -> UpdatedReferenceCmds/1
  ReferenceValueServerCmds/1 -> Bus Assignment/1
  EstimatedVal/1 -> Bus Selector1/1
  Bus Selector1/1 -> Terminator1/1  "<X>"
  Bus Selector1/2 -> Terminator2/1  "<Y>"
  Bus Selector1/3 -> Terminator3/1  "<Z>"
  Bus Selector1/4 -> Terminator4/1  "<yaw>"
  Bus Selector1/5 -> Terminator5/1  "<pitch>"
  Bus Selector1/6 -> Terminator6/1  "<roll>"
  Delay3/1 -> Add1/2
  Add1/1 -> Delay3/1, Mux1/2  "yValue"
  Delay4/1 -> Add2/2
  Add2/1 -> Delay4/1, Mux1/1  "xValue"
  Mux1/1 -> Data Type Conversion1/1
  Switch5/1 -> Mux1/3
  Data Type Conversion1/1 -> Bus Assignment/2
  Switch Case1/2 -> Switch Case Action Subsystem7/Action
  Switch Case1/3 -> Switch Case Action Subsystem6/Action
  Switch Case Action Subsystem7/1(Out1) -> Merge/1
  Switch Case Action Subsystem6/1(Out1) -> Merge/2
  Merge/1 -> Delay6/1, Switch3/3, Switch/3
  Switch Case Action Subsystem3/1(Out1) -> Merge1/3
  Switch Case/2 -> Switch Case Action Subsystem4/Action
  Switch Case Action Subsystem4/1(Out1) -> Merge1/2
  Switch Case/3 -> Switch Case Action Subsystem3/Action
  Switch Case/1 -> Switch Case Action Subsystem5/Action
  Delay8/1 -> Switch Case Action Subsystem5/1(In1)
  Switch Case Action Subsystem5/1(Out1) -> Merge1/1
  Switch Case Action Subsystem2/1(Out1) -> Merge/3
  Switch Case1/1 -> Switch Case Action Subsystem2/Action
  Delay7/1 -> Switch Case Action Subsystem2/1(In1)
  Constant2/1 -> Product1/2
  Product1/1 -> Switch Case Action Subsystem4/1(In1)
  Product2/1 -> Switch Case Action Subsystem3/1(In1)
  Constant5/1 -> Product2/2
  Product/1 -> Switch Case Action Subsystem7/1(In1)
  Constant/1 -> Product/2
  Product3/1 -> Switch Case Action Subsystem6/1(In1)
  Constant1/1 -> Product3/2
  PD_up/1 -> Gain2/1
  PD_down/1 -> Gain5/1
  PD_left/1 -> Gain6/1
  PD_right/1 -> Gain7/1
  Gain/1 -> Scope/2, Add1/1
  Gain1/1 -> Scope/1, Add2/1
  Gain2/1 -> Scope1/1, Product1/1  "PID_ue"
  Gain5/1 -> Product2/1
  Gain6/1 -> Product/1
  Gain7/1 -> Scope1/4, Product3/1
  sayu/1 -> 最初の動きと4分割出力_左右/1(In1)
  外枠左右/1 -> 最初の動きと4分割出力_左右/2(外枠左右)
  zyouge/1 -> 最初の動きと4分割出力_上下/1(In1)
  外枠上下/1 -> 最初の動きと4分割出力_上下/2(外枠上下(0,5,3,4))
  最初の動きと4分割出力_上下/1(Out1) -> Threshold for each pixel4/1, Switch Case/1  "上下分岐"
  角検知_左右(1,2)/1 -> Data Type Conversion/1
  Switch Case2/1 -> Switch Case Action Subsystem8/Action
  Switch Case2/2 -> Switch Case Action Subsystem9/Action
  Switch Case2/3 -> Switch Case Action Subsystem10/Action
  Constant3/1 -> Switch Case Action Subsystem9/1(In1)
  Constant4/1 -> Switch Case Action Subsystem10/1(In1)
  Delay2/1 -> Gain8/1
  Gain8/1 -> Switch Case Action Subsystem8/1(In1)
  Switch Case Action Subsystem8/1(Out1) -> Merge2/1
  Switch Case Action Subsystem9/1(Out1) -> Merge2/2
  Switch Case Action Subsystem10/1(Out1) -> Merge2/3
  Merge2/1 -> Switch/1
  Data Type Conversion/1 -> Switch Case2/1
  Switch Case3/2 -> Switch Case Action Subsystem12/Action
  Switch Case Action Subsystem12/1(Out1) -> Merge3/2
  Constant6/1 -> Switch Case Action Subsystem12/1(In1)
  Gain3/1 -> Switch Case Action Subsystem11/1(In1)
  Switch Case Action Subsystem11/1(Out1) -> Merge3/1
  Switch Case3/3 -> Switch Case Action Subsystem1/Action
  Delay5/1 -> Gain3/1
  Data Type Conversion2/1 -> Scope1/3, Switch Case3/1  "角検知_上下"
  角の動きするか(0,1)/1 -> AND/2, AND1/1, Switch2/2, Switch3/2
  Merge3/1 -> Switch1/1
  Merge1/1 -> Switch2/3, Delay1/1, Switch1/3
  角検知_上下(3,4)/1 -> Data Type Conversion2/1
  Switch Case Action Subsystem1/1(Out1) -> Merge3/3
  Constant7/1 -> Switch Case Action Subsystem1/1(In1)
  Switch Case3/1 -> Switch Case Action Subsystem11/Action
  Switch1/1 -> Threshold for each pixel1/1, Scope1/5, zyouge_out/1, Switch2/1, Gain1/1  "上下"
  Switch Case/4 -> Switch Case Action Subsystem13/Action
  Delay1/1 -> Switch Case Action Subsystem13/1(In1)
  Switch Case Action Subsystem13/1(Out1) -> Merge1/4
  Switch Case/5 -> Switch Case Action Subsystem14/Action
  Constant8/1 -> Switch Case Action Subsystem14/1(In1)
  Switch Case Action Subsystem14/1(Out1) -> Merge1/5
  Switch Case/6 -> Switch Case Action Subsystem15/Action
  Constant9/1 -> Switch Case Action Subsystem15/1(In1)
  Switch Case Action Subsystem15/1(Out1) -> Merge1/6
  Switch Case1/4 -> Switch Case Action Subsystem16/Action
  Switch Case1/5 -> Switch Case Action Subsystem17/Action
  Switch Case1/6 -> Switch Case Action Subsystem18/Action
  Switch Case Action Subsystem16/1(Out1) -> Merge/4
  Switch Case Action Subsystem17/1(Out1) -> Merge/5
  Switch Case Action Subsystem18/1(Out1) -> Merge/6
  Delay6/1 -> Switch Case Action Subsystem16/1(In1)
  Constant10/1 -> Switch Case Action Subsystem17/1(In1)
  Constant11/1 -> Switch Case Action Subsystem18/1(In1)
  最初の動きと4分割出力_左右/1(Out1) -> Scope1/2, Threshold for each pixel2/1, Switch Case1/1
  Switch2/1 -> Delay8/1
  Switch3/1 -> Delay7/1
  zValue/1 -> Switch5/3
  zValue2/1 -> Switch5/1
  Switch Case1/7 -> Switch Case Action Subsystem19/Action
  Constant12/1 -> Switch Case Action Subsystem19/1(In1)
  Switch Case Action Subsystem19/1(Out1) -> Merge/7
  Switch Case/7 -> Switch Case Action Subsystem20/Action
  Constant13/1 -> Switch Case Action Subsystem20/1(In1)
  Switch Case Action Subsystem20/1(Out1) -> Merge1/7
  Z軸/1 -> Switch5/2
  Constant14/1 -> Switch Case Action Subsystem21/1(In1)
  Constant15/1 -> Switch Case Action Subsystem22/1(In1)
  Switch Case/8 -> Switch Case Action Subsystem21/Action
  Switch Case Action Subsystem21/1(Out1) -> Merge1/8
  Switch Case Action Subsystem22/1(Out1) -> Merge1/9
  Constant16/1 -> Switch Case Action Subsystem23/1(In1)
  Switch Case1/9 -> Switch Case Action Subsystem24/Action
  Constant17/1 -> Switch Case Action Subsystem24/1(In1)
  Switch Case1/8 -> Switch Case Action Subsystem23/Action
  Switch Case Action Subsystem23/1(Out1) -> Merge/9
  Switch Case Action Subsystem24/1(Out1) -> Merge/8
  Switch Case/9 -> Switch Case Action Subsystem22/Action
  Threshold for each pixel2/1 -> AND/1
  AND/1 -> Switch/2
  Switch4/1 -> Delay5/1
  Threshold for each pixel1/1 -> Switch4/2
  Constant18/1 -> Switch4/1
  Constant19/1 -> Switch4/3
  Switch6/1 -> Delay2/1
  Constant20/1 -> Switch6/1
  Constant21/1 -> Switch6/3
  Switch/1 -> Threshold for each pixel3/1, Scope1/6, sayu_out/1, Gain/1, Switch3/1  "上下"
  Threshold for each pixel3/1 -> Switch6/2
  Threshold for each pixel4/1 -> AND1/2
  AND1/1 -> Switch1/2

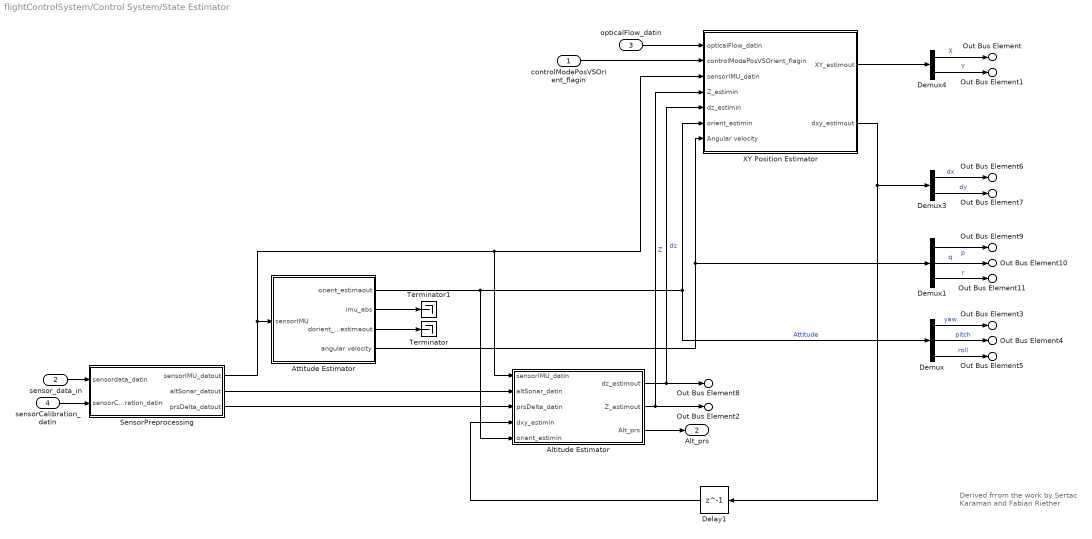
== system flightControlSystem/Control System/State Estimator ==
  note: Derived frrom the work by Sertac
      | Karaman and Fabian Riether
  controlModePosVSOrient_flagin : Inport  OutDataTypeStr=boolean
  sensor_data_in : Inport  Port=2
  opticalFlow_datin : Inport  Port=3
  sensorCalibration_datin : Inport  Port=4
  Altitude Estimator : Subsystem
  Attitude Estimator : Subsystem
  Delay1 : Delay  DelayLength=1  InitialCondition=0
  Demux : Demux  Outputs=3
  Demux1 : Demux  Outputs=3
  Demux3 : Demux  Outputs=2
  Demux4 : Demux  Outputs=2
  SensorPreprocessing : Subsystem
  Terminator : Terminator
  Terminator1 : Terminator
  XY Position Estimator : Subsystem
  Out Bus Element : Outport  VectorParamsAs1DForOutWhenUnconnected=off  PortName=states_estim  Element=X
  Out Bus Element1 : Outport  VectorParamsAs1DForOutWhenUnconnected=off  PortName=states_estim  Element=Y
  Out Bus Element2 : Outport  VectorParamsAs1DForOutWhenUnconnected=off  PortName=states_estim  Element=Z
  Out Bus Element3 : Outport  VectorParamsAs1DForOutWhenUnconnected=off  PortName=states_estim  Element=yaw
  Out Bus Element4 : Outport  VectorParamsAs1DForOutWhenUnconnected=off  PortName=states_estim  Element=pitch
  Out Bus Element5 : Outport  VectorParamsAs1DForOutWhenUnconnected=off  PortName=states_estim  Element=roll
  Out Bus Element6 : Outport  VectorParamsAs1DForOutWhenUnconnected=off  PortName=states_estim  Element=dx
  Out Bus Element7 : Outport  VectorParamsAs1DForOutWhenUnconnected=off  PortName=states_estim  Element=dy
  Out Bus Element8 : Outport  VectorParamsAs1DForOutWhenUnconnected=off  PortName=states_estim  Element=dz
  Out Bus Element9 : Outport  VectorParamsAs1DForOutWhenUnconnected=off  PortName=states_estim  Element=p
  Out Bus Element10 : Outport  VectorParamsAs1DForOutWhenUnconnected=off  PortName=states_estim  Element=q
  Out Bus Element11 : Outport  VectorParamsAs1DForOutWhenUnconnected=off  PortName=states_estim  Element=r
  Alt_prs : Outport  Port=2  VectorParamsAs1DForOutWhenUnconnected=off
  wires:
  XY Position Estimator/2(dxy_estimout) -> Demux3/1, Delay1/1
  Demux1/3 -> Out Bus Element11/1  "r"
  Demux/3 -> Out Bus Element5/1  "roll"
  Demux4/2 -> Out Bus Element1/1  "Y"
  XY Position Estimator/1(XY_estimout) -> Demux4/1
  Attitude Estimator/2(imu_abs) -> Terminator1/1
  Attitude Estimator/4(angular velocity) -> XY Position Estimator/7(Angular velocity), Demux1/1
  sensor_data_in/1 -> SensorPreprocessing/1(sensordata_datin)
  opticalFlow_datin/1 -> XY Position Estimator/1(opticalFlow_datin)
  Demux4/1 -> Out Bus Element/1  "X"
  SensorPreprocessing/1(sensorIMU_datout) -> Attitude Estimator/1(sensorIMU), XY Position Estimator/3(sensorIMU_datin), Altitude Estimator/1(sensorIMU_datin)
  SensorPreprocessing/3(prsDelta_datout) -> Altitude Estimator/3(prsDelta_datin)
  Demux3/2 -> Out Bus Element7/1  "dy"
  SensorPreprocessing/2(altSonar_datout) -> Altitude Estimator/2(altSonar_datin)
  Altitude Estimator/1(dz_estimout) -> XY Position Estimator/5(dz_estimin), Out Bus Element8/1  "dz"
  Altitude Estimator/2(Z_estimout) -> XY Position Estimator/4(Z_estimin), Out Bus Element2/1  "Z"
  Demux1/1 -> Out Bus Element9/1  "p"
  Demux3/1 -> Out Bus Element6/1  "dx"
  Attitude Estimator/3(dorient_estimaout) -> Terminator/1
  Demux/2 -> Out Bus Element4/1  "pitch"
  controlModePosVSOrient_flagin/1 -> XY Position Estimator/2(controlModePosVSOrient_flagin)
  Attitude Estimator/1(orient_estimaout) -> XY Position Estimator/6(orient_estimin), Demux/1, Altitude Estimator/5(orient_estimin)  "Attitude"
  Demux/1 -> Out Bus Element3/1  "yaw"
  Delay1/1 -> Altitude Estimator/4(dxy_estimin)
  Demux1/2 -> Out Bus Element10/1  "q"
  sensorCalibration_datin/1 -> SensorPreprocessing/2(sensorCalibration_datin)
  Altitude Estimator/3(Alt_prs) -> Alt_prs/1
